simulink model "Accelerator"  (R2022b)
settings: Solver=FixedStepDiscrete  StartTime=0.0  StopTime=10  FixedStep=0.005  RelTol=1e-3  EnableMultiTasking=on
PreLoadFcn:
  | try, model_open; catch, disp('Error occurred while executing model pre-load callback: model_open.m'); disp('Please assure that the MATLAB working directory is set to the model directory before opening.'); end
InitFcn:
  | try, model_open; catch, end
undefined symbols (not defined in the file): GCM, raptor_get_safe_string, raptor_xcp_function
libraries: Raptor_lib x134, simulink x14, Blocks_Library x2, simulink_extras x1
(part 1 of 3)
CloseFcn:
  | try, model_close; catch, end
settings Model: Raptor_Target=GCM-1793-196-1503  Raptor_Calloc=NonVolatile (EEPROM)  RaptorUIDSize=4  RaptorBuildNum=19  Raptor_ecuaddr=11  RaptorFaultManager=Standard  RaptorFaultManagerAddXYCounts=1  Raptor_IsLiteMode=0  Creator=Ben  LastModifiedBy=Jhon
settings SolverCC: AlgebraicLoopSolver=TrustRegion
settings DataIOCC: LimitDataPoints=on  SaveFormat=Array  SignalLoggingSaveFormat=ModelDataLogs  ReturnWorkspaceOutputs=off
settings OptimizationCC: DefaultParameterBehavior=Inlined  ExpressionDepthLimit=2147483647  InitFltsAndDblsToZero=on  LifeSpan=1  EfficientTunableParamExpr=on
settings DebuggingCC: SolverPrmCheckMsg=warning  InheritedTsInSrcMsg=none  ParameterPrecisionLossMsg=none  FcnCallInpInsideContextMsg=warning  UnconnectedInputMsg=warning  UnconnectedOutputMsg=warning  UnconnectedLineMsg=warning  StateNameClashWarn=warning  SFUnexpectedBacktrackingDiag=warning  SFNoUnconditionalDefaultTransitionDiag=warning  SFExecutionAtInitializationDiag=none  SFMachineParentedDataDiag=warning  ArithmeticOperatorsInVariantConditions=warning
settings HardwareCC: ProdBitPerPointer=32  ProdBitPerSizeT=32  ProdBitPerPtrDiffT=32  ProdLargestAtomicFloat=None  ProdWordSize=32  ProdHWDeviceType=Infineon->TriCore  TargetIntDivRoundTo=Zero  TargetEndianess=LittleEndian  ProdEqTarget=off
settings ModelReferenceCC: EnableRefExpFcnMdlSchedulingChecks=on  PropagateSignalLabelsOutOfModel=off
settings SFSimCC: SimUseLocalCustomCode=off  MATLABDynamicMemAlloc=off  CustomCodeUndefinedFunction=UseInterfaceOnly
settings RTWCC: Description=Raptor (tm)  SystemTargetFile=raptor.tlc  GenCodeOnly=on  MakeCommand=raptor_make_rtw  TemplateMakefile=raptor.tmf  RTWUseLocalCustomCode=off
settings CodeAppCC: IgnoreCustomStorageClasses=off  MaxIdLength=100  CustomSymbolStrType=$N$R$M  StateflowObjectComments=on  InternalIdentifier=Classic
settings STFCustomTargetCC: CodeReplacementLibrary=GCM196-specific  GenerateSampleERTMain=on  ModelReferenceCompliant=off  CombineOutputUpdateFcns=on  ERTCustomFileBanners=on  SupportContinuousTime=off  SupportNonInlinedSFcns=off  RemoveResetFunc=on  MATLABClassNameForMDSCustomization=Simulink.SoftwareTarget.ERTCustomization  SystemTargetFile=raptor.tlc
settings ERTTargetCC: CodeReplacementLibrary=GCM196-specific  MultiwordLength=2048  GenerateSampleERTMain=on  ModelReferenceCompliant=off  ParMdlRefBuildCompliant=off  CompOptLevelCompliant=off  ConcurrentExecutionCompliant=off  ModelStepFunctionPrototypeControlCompliant=off  CPPClassGenCompliant=off  UseToolchainInfoCompliant=off  ExtModeMexFile=noextcomm  InlinedParameterPlacement=NonHierarchical  ERTCustomFileTemplate=example_file_process.tlc  ConvertIfToSwitch=off  SuppressUnreachableDefaultCases=off
settings ConfigComp: CovMetricSettings=dw  CovSaveCumulativeToWorkspaceVar=on  CovSaveSingleToWorkspaceVar=on  CovExternalEMLEnable=off  CovSFcnEnable=off

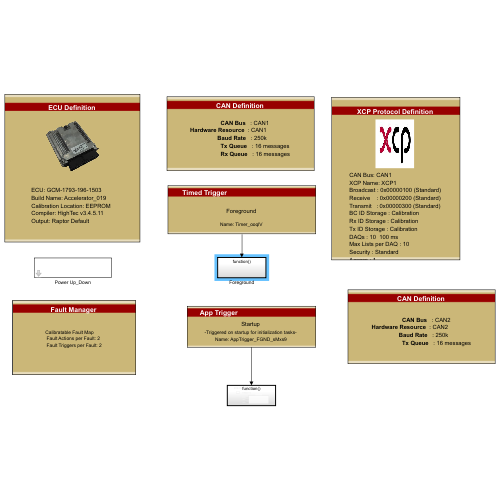
[thumbnail: Simulink's stored preview of the top-level diagram]
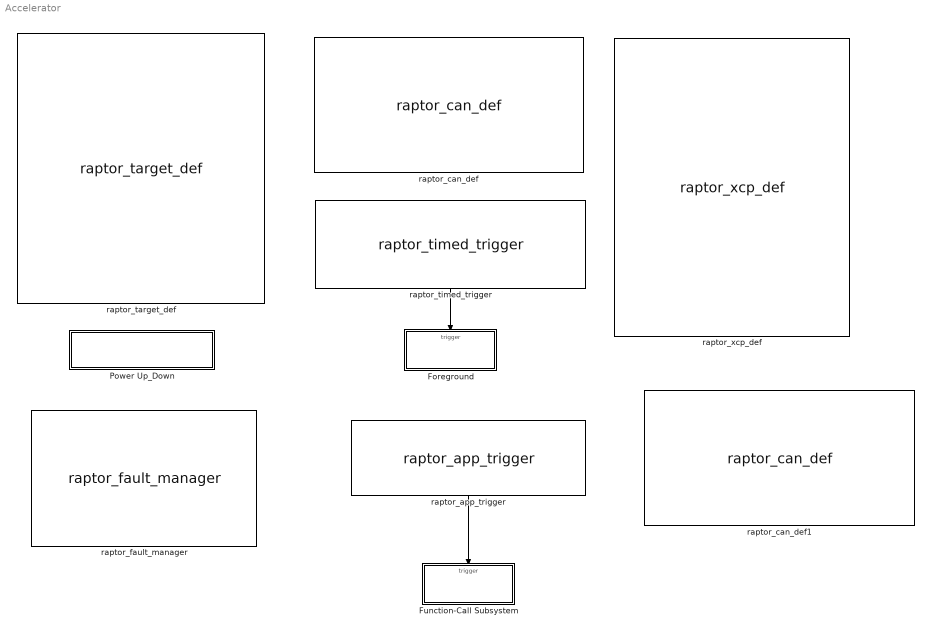
== system Accelerator ==
  Foreground : Subsystem  TreatAsAtomicUnit=on
      settings: RTWSystemCode=Nonreusable function
  Function-Call Subsystem : Subsystem  TreatAsAtomicUnit=on
  Power Up_Down : Subsystem  mask{group='Diagnostics | Power Up_Down'}
  raptor_app_trigger : Raptor_lib/Triggers/raptor_app_trigger  triggerValues=Startup|Shutdown|SafetyMonitor  trigger=Startup  inherited=0  alwaysEnabled=1  triggerPriority=1  triggerName=FGND_sMxs9  allowInline=0
      settings: SourceProductName=Raptor
  raptor_can_def : Raptor_lib/CAN/raptor_can_def  canBus='CAN1'  resourceValues=CAN1|CAN2|CAN3|(None)  resource=CAN1  baudRateValues=125k|250k|500k|1000k  baudRate=250k  enable_baud_rate_config='RAPTOR MASK DEFAULT'  sim_func_name='RAPTOR MASK DEFAULT'  createButton=[]  txQueueSize=16  rxQueueSize=16
      settings: SourceProductName=Raptor
  raptor_can_def1 : Raptor_lib/CAN/raptor_can_def  canBus='CAN2'  resourceValues=CAN1|CAN2|CAN3|(None)  resource=CAN2  baudRateValues=125k|250k|500k|1000k  baudRate=250k  enable_baud_rate_config='RAPTOR MASK DEFAULT'  sim_func_name='RAPTOR MASK DEFAULT'  createButton=[]  txQueueSize=16  rxQueueSize=16
      settings: SourceProductName=Raptor
  raptor_fault_manager : Raptor_lib/Faults/raptor_fault_manager  button=0  managerTypeValues=Standard|OBD  managerType=Standard  cyclesToHeal=3  cyclesToClear=40  addXYCounts=1  calFaultMap=1  minFaultActions=2  minFaultTriggers=2  calAccessValues=4|3|2|1  calAccess=4  calFunction='System | FaultManager'  initMap=struct('managerType', 'Standard','actionMap', {{}},'triggerMap', {{}})  exportFilePath='C:\'  exportFileName='FaultMapExport_01.csv'
      settings: SourceProductName=Raptor
  raptor_target_def : Raptor_lib/Configuration/raptor_target_def  targetValues=BCM-5646-48-1404|DISP-VC128-1901|DISP-VC320L-1402|DISP-VC320-1204|DISP-VC800-1402|DISP-VC500-1904|DISP-VC700-2003|DISP-VC300R-2004|GCM-5634M-070-1459|GCM-5634M-070-1559|GCM-5634M-070-1562|ECM-1793-196-1503|GCM-1793-196-1503|GCM-5605B-048-1906|GCM-5605B-048-2104|GCM-5607B-80-1901|GCM-5607B-80-1903|GCM-5607B-80-2001|RCM-5743R-080-2005|RCM-5743R-080-2106|RCM-5743R-080-2203|UAS-5743R-047-2102|UAS-5743R-047-2107|GCM-5746R-048-1902|RCM-58NN-112-2007|RCM-58NN-112-2103|RCM-58NN-112-2202|HCM-5604-36-1303|HCM-5604-36-1702  target=GCM-1793-196-1503  simpack=0  simulator=0  heap=4*1024  stack=2*1024  fgndStack=3*1024  bgndStack=2*1024  idleStack=1024  intStack=1536  sdStack=1024  appStack=1024  ecuaddr=11  uds_server_addr_ext=0  uds_server_addr=hex2dec('600')  uds_client_addr=hex2dec('650')  callocValues=Constant (FLASH)|NonVolatile (EEPROM)  calloc=NonVolatile (EEPROM)  compilerValues=HighTec v3.4.5.11  compiler=HighTec v3.4.5.11  setFileName=0  exeName=[raptor_get_safe_string(bdroot) '_']  addBuildNum=1  minVerChars=3  extraOutput=0  buildLocationValues=Raptor Default|Model Directory|User Defined  buildLocation=Raptor Default  exeLocation=''  exeFileButton=0  a2lLocation=''  a2lFileButton=0  rpgLocation=''  rpgFileButton=0
      settings: SourceProductName=Raptor
  raptor_timed_trigger : Raptor_lib/Triggers/raptor_timed_trigger  triggerValues=Foreground|Foregroundx2|Foregroundx5|Foregroundx10|Foregroundx20|Background|Backgroundx2|Backgroundx5|Backgroundx10|Backgroundx20|Second|Minute|Task_1ms  trigger=Foreground  inherited=0  alwaysEnabled=1  triggerPriority=0  triggerName=ooqlV
      settings: SourceProductName=Raptor
  raptor_xcp_def : Raptor_lib/Configuration/raptor_xcp_def  XCPname='XCP1'  canBus='CAN1'  bcID=hex2dec('100')  bcID_TypeValues=Standard|Extended  bcID_Type=Standard  rxID=hex2dec('200')  rxID_TypeValues=Standard|Extended  rxID_Type=Standard  txID=hex2dec('300')  txID_TypeValues=Standard|Extended  txID_Type=Standard  daqRates=[10 100]  numODTs=10  genCANAPE=0  genVISION=0  securityValues=Standard|None|Custom User Defined  security=Standard  dllName=raptor_XCPSecurity.dll  accessValues=4|3|2|1  access=1  bcStorageValues=Constant (FLASH)|NonVolatile (EEPROM)|FixedNonVolatile (EEPROM)|Volatile (RAM)|Calibration  bcStorage=Calibration  txStorageValues=Constant (FLASH)|NonVolatile (EEPROM)|FixedNonVolatile (EEPROM)|Volatile (RAM)|Calibration  txStorage=Calibration  rxStorageValues=Constant (FLASH)|NonVolatile (EEPROM)|FixedNonVolatile (EEPROM)|Volatile (RAM)|Calibration  rxStorage=Calibration
      settings: SourceProductName=Raptor
  wires:
  raptor_app_trigger/1 -> Function-Call Subsystem/Trigger
  raptor_timed_trigger/1 -> Foreground/Trigger
